simulink model "boostpfc"  (R2014a)
settings: Solver=ode23tb  StartTime=0.0  StopTime=0.4  MaxStep=0.01  RelTol=1e-3
libraries: powerlib x22, powerlib_meascontrol x5
settings Model: Creator=hp  LastModifiedBy=hp
settings SolverCC: SolverResetMethod=Robust

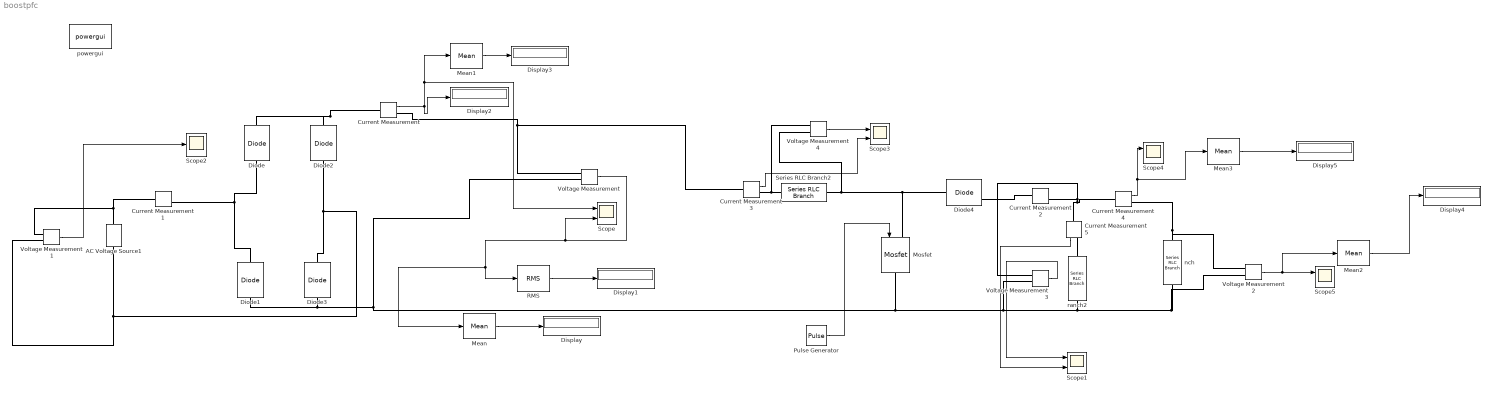
== system boostpfc ==
  AC Voltage Source1 : powerlib/Electrical Sources/AC Voltage Source  Amplitude=230  Phase=0  Frequency=50  SampleTime=0  Measurements=None
  Current Measurement{,1..5} (6 alike) : powerlib/Measurements/Current Measurement  PhasorSimulation=off  OutputType=Complex  PSBequivalent=0
  Diode{,1..3} (4 alike) : powerlib/Power Electronics/Diode  Ron=0.001  Lon=0  Vf=0.8  IC=0  UseSnubber=off  Rs=500  Cs=250e-9  Measurements=off
  Diode4 : powerlib/Power Electronics/Diode  Ron=0.001  Lon=0  Vf=0.8  IC=0  UseSnubber=off  Rs=500  Cs=250e-9  Measurements=on
  Display{,1..5} (6 alike) : Display
  Mean : powerlib_meascontrol/Measurements/Mean  Freq=50  Vinit=0  Ts=0
  Mean1 : powerlib_meascontrol/Measurements/Mean  Freq=60  Vinit=0  Ts=0
  Mean2 : powerlib_meascontrol/Measurements/Mean  Freq=50  Vinit=0  Ts=0
  Mean3 : powerlib_meascontrol/Measurements/Mean  Freq=50  Vinit=0  Ts=0
  Mosfet : powerlib/Power Electronics/Mosfet  Ron=0.1  Lon=0  Rd=0.01  Vfd=0  IC=0  Rs=1e5  Cs=inf  Measurements=off
  Pulse Generator : DiscretePulseGenerator  PulseType=Time based  Period=1/2000  PulseWidth=63.4
  RMS : powerlib_meascontrol/Measurements/RMS  TrueRMS=on  Freq=60  RMSInit=120  Ts=0
  Scope{,1,3..5} (5 alike) : Scope  NumInputPorts=2
      Scope settings: TimeRange=1.199999999999999  YMin=0~-5  YMax=250~5  SaveName=scopeLoggedData
      Scope1 settings: YMin=-5~-5  YMax=5~5
      Scope3 settings: YMin=144.67~191.5  YMax=144.679~192.5
      Scope4 settings: YMin=-5~-5  YMax=5~5  SaveName=ScopeData4
      Scope5 settings: YMin=1.0035~-5  YMax=1.0135~5  SaveName=ScopeData3
  Scope2 : Scope
      settings: SaveName=ScopeData2
  Series RLC Branch2 : powerlib/Elements/Series RLC Branch  LConnTagsString=__new0  RConnTagsString=__new0  BranchType=L  Resistance=1  Inductance=12.3e-3  SetiL0=off  InitialCurrent=0  Capacitance=1e-6  Setx0=off  InitialVoltage=0  Measurements=None
  Voltage Measurement{,1..4} (5 alike) : powerlib/Measurements/Voltage Measurement  PhasorSimulation=off  OutputType=Complex  PSBequivalent=0
  nch : powerlib/Elements/Series RLC Branch  LConnTagsString=__new0  RConnTagsString=__new0  BranchType=R  Resistance=1600  Inductance=1e-3  SetiL0=off  InitialCurrent=0  Capacitance=1e-6  Setx0=off  InitialVoltage=0  Measurements=None
  powergui : powerlib/powergui  Priority=1  SimulationMode=Continuous  SolverType=Tustin  SampleTime=50e-6  frequency=60  SPID=off  DisableSnubberDevices=off  DisableRonSwitches=off  DisableVfSwitches=off  SwTol=0  Interpol=off  DisplayEquations=off  Ts=0  methode=off  frequencyindice=50  Pbase=100e6  ErrMax=1e-4  Iterations=50  UnitsV=kV  UnitsW=MW  FunctionMessages=off  echomessages=off  HookPort=off  EnableUseOfTLC=off  x0status=blocks  RestoreLinks=warning  ResistiveCurrentMeasurement=off  Frange=[0:2:500]  Ylog=off  Xlog=on  ShowGrid=off  save=off  variable=ZData  structure=0  ZoomFFT=off  StartTime=0.0  cycles=1  DisplayStyle=1  fundamental=60  FreqAxis=off  MaxFrequency=1000  frequencyindicesteady=1  RmsSteady=1  display=off
  ranch2 : powerlib/Elements/Series RLC Branch  LConnTagsString=__new0  RConnTagsString=__new0  BranchType=C  Resistance=1  Inductance=1e-3  SetiL0=off  InitialCurrent=0  Capacitance=0.1585e-6  Setx0=off  InitialVoltage=0  Measurements=None
  wires:
  Voltage Measurement/1 -> Scope/2, Mean/1, RMS/1
  RMS/1 -> Display1/1
  Mean/1 -> Display/1
  Current Measurement/1 -> Display2/1, Scope/1, Mean1/1
  Mean1/1 -> Display3/1
  Voltage Measurement4/1 -> Scope3/1
  Pulse Generator/1 -> Mosfet/1
  Voltage Measurement3/1 -> Scope1/1
  Current Measurement5/1 -> Scope1/2
  Current Measurement4/1 -> Mean3/1, Scope4/1
  Voltage Measurement2/1 -> Mean2/1, Scope5/1
  Current Measurement3/1 -> Scope3/2
  Voltage Measurement1/1 -> Scope2/1
  Mean2/1 -> Display4/1
  Mean3/1 -> Display5/1
  connections:
  Diode/LConn1 -- Current Measurement1/RConn1 -- Diode1/RConn1
  Diode/RConn1 -- Current Measurement/LConn1 -- Diode2/RConn1
  Diode3/RConn1 -- AC Voltage Source1/LConn1 -- Voltage Measurement1/LConn2 -- Diode2/LConn1
  ranch2/LConn1 -- Voltage Measurement2/LConn2 -- nch/RConn1 -- Voltage Measurement/LConn2 -- Diode3/LConn1 -- Diode1/LConn1 -- Mosfet/RConn1 -- Voltage Measurement3/LConn2
  Voltage Measurement/LConn1 -- Current Measurement3/LConn1 -- Current Measurement/RConn1
  Current Measurement1/LConn1 -- Voltage Measurement1/LConn1 -- AC Voltage Source1/RConn1
  Current Measurement3/RConn1 -- Voltage Measurement4/LConn1 -- Series RLC Branch2/LConn1
  Series RLC Branch2/RConn1 -- Diode4/LConn1 -- Mosfet/LConn1 -- Voltage Measurement4/LConn2
  Current Measurement2/RConn1 -- Current Measurement5/LConn1 -- Current Measurement4/LConn1 -- Voltage Measurement3/LConn1
  nch/LConn1 -- Current Measurement4/RConn1 -- Voltage Measurement2/LConn1
  Current Measurement5/RConn1 -- ranch2/RConn1
  Diode4/RConn1 -- Current Measurement2/LConn1
